simulink library "alfa_wall_out"  (R2018b)
settings: Solver=ode45  StartTime=0.0  StopTime=10.0  RelTol=1e-3  EnableMultiTasking=on
libraries: carnot x2
settings Model: Creator=lena.frank  LastModifiedBy=drhf
settings DataIOCC: LimitDataPoints=on  SaveFormat=Array  SignalLoggingSaveFormat=ModelDataLogs
settings OptimizationCC: ExpressionDepthLimit=2147483647  LifeSpan=inf
settings DebuggingCC: UnderspecifiedInitializationDetection=Classic  MergeDetectMultiDrivingBlocksExec=none  SolverPrmCheckMsg=warning  FcnCallInpInsideContextMsg=warning  StateNameClashWarn=warning  SFUnexpectedBacktrackingDiag=warning  SFNoUnconditionalDefaultTransitionDiag=warning  SFExecutionAtInitializationDiag=none
settings HardwareCC: ProdBitPerPointer=32  ProdBitPerSizeT=32  ProdBitPerPtrDiffT=32  ProdLargestAtomicFloat=None  ProdIntDivRoundTo=Undefined  ProdEndianess=Unspecified  ProdWordSize=32  ProdHWDeviceType=32-bit Generic
settings ModelReferenceCC: PropagateSignalLabelsOutOfModel=off
settings SFSimCC: SimUseLocalCustomCode=off
settings RTWCC: RTWUseLocalCustomCode=off
settings CodeAppCC: StateflowObjectComments=on
settings GRTTargetCC: TargetLangStandard=C89/C90 (ANSI)  GeneratePreprocessorConditionals=Disable all  CombineOutputUpdateFcns=off  GRTInterface=on
settings ConfigComp: CovMetricSettings=dw  CovHtmlReporting=on  CovSaveCumulativeToWorkspaceVar=on  CovSaveSingleToWorkspaceVar=on  CovExternalEMLEnable=off

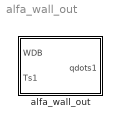
== system alfa_wall_out ==
  alfa_wall_out : Subsystem  mask(ALFA){pos=0, absorption_out=0.4, emission_out=0.7, wallsurface=1}
      mask prompts: pos "Azimut (south = 0, east = -90) in degrees"; absorption_out "Solar absorption outside (0..1)"; emission_out "Longwave emissivity of surface (0..1)"; wallsurface "Wall surface in m²"
      mask help:
      | Convective and radiative HEAT TRANSFER at the WEATHER EXPOSED SURFACE of an OUTER WALL.
      |
      | [W*] : modified weather data, adapted to height over ground,
      | Ts : temperature of outdoor wall surface, °C,
      | qdots : specific heat flow into wall / window construction, W/m^2.
      mask init:
      | if length(pos) == 1
      |     pos = [90  pos 0]; % pos is [inclination azimut rotation]
      | end
      mask Help: web(fullfile(path_carnot('help'),'alfa_wall_out.html'),'-helpbrowser')

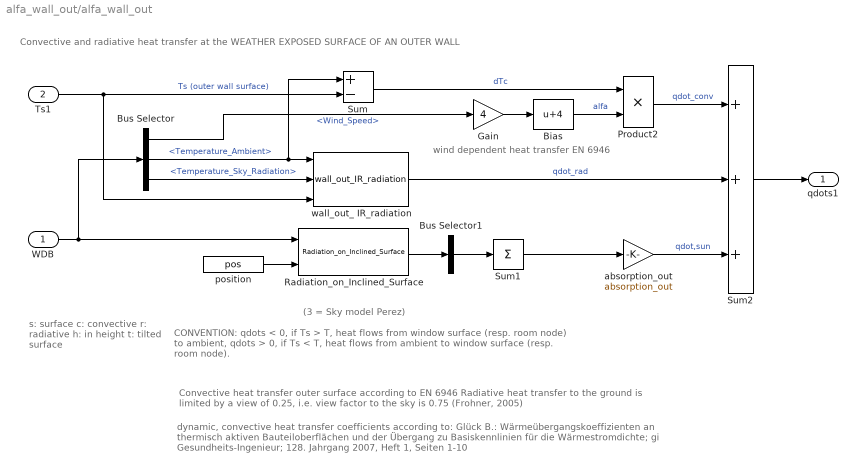
== system alfa_wall_out/alfa_wall_out ==
  note: (3 = Sky model Perez)
  note: wind dependent heat transfer EN 6946
  note: CONVENTION:
      | qdots < 0, if Ts > T, heat flows from window surface (resp. room node) to ambient,
      | qdots > 0, if Ts < T, heat flows from ambient to window surface (resp. room node).
  note: s: surface
      | c: convective
      | r: radiative
      | h: in height
      | t: tilted surface
  note: Convective and radiative heat transfer at the WEATHER EXPOSED SURFACE OF AN OUTER WALL
  note: Convective heat transfer outer surface according to EN 6946
      | Radiative heat transfer to the ground is limited by a view of 0.25, i.e. view factor to the sky is 0.75 (Frohner, 2005)
  note: dynamic, convective heat transfer coefficients according to: Glück B.: Wärmeübergangskoeffizienten an thermisch aktiven Bauteiloberflächen
      | und der Übergang zu Basiskennlinien für die Wärmestromdichte; gi Gesundheits-Ingenieur; 128. Jahrgang 2007, Heft 1, Seiten 1-10
  WDB : Inport
  Ts1 : Inport  Port=2
  Bias : Bias  Bias=4
  Bus Selector : BusSelector  OutputSignals=Wind_Speed,Temperature_Ambient,Temperature_Sky_Radiation
  Bus Selector1 : BusSelector  OutputSignals=Solar_Radiation_direct_surface,Solar_Radiation_diffuse_surface  OutputAsBus=on
  Gain : Gain  Gain=4
  Product2 : Product  SaturateOnIntegerOverflow=on  RndMeth=Zero  InputSameDT=on  OutDataTypeStr=Inherit: Same as first input
  Radiation_on_Inclined_Surface : carnot/Weather/Radiation_on_Inclined_Surface  sky=Perez 1990  reflect=0.2
      settings: SourceProductName=Carnot
  Sum : Sum  Inputs=+-  SaturateOnIntegerOverflow=on  InputSameDT=on  OutDataTypeStr=Inherit: Same as first input
  Sum1 : Sum  Inputs=1  SaturateOnIntegerOverflow=on  InputSameDT=on  OutDataTypeStr=Inherit: Same as first input
  Sum2 : Sum  Inputs=+++  SaturateOnIntegerOverflow=on  InputSameDT=on  OutDataTypeStr=Inherit: Same as first input
  absorption_out : Gain  Gain=absorption_out  SaturateOnIntegerOverflow=on  OutDataTypeStr=Inherit: Same as input  ParamDataTypeStr=Inherit: Same as input
  position : Constant  Value=pos
  wall_out_ IR_radiation : carnot/Basic/Heat_Transfer/wall_out_IR_radiation  SystemSampleTime=-1
      settings: SourceProductName=Carnot
  qdots1 : Outport
  wires:
  position/1 -> Radiation_on_Inclined_Surface/2
  Radiation_on_Inclined_Surface/1 -> Bus Selector1/1
  Bus Selector1/1 -> Sum1/1
  wall_out_ IR_radiation/1 -> Sum2/2  "qdot_rad"
  Product2/1 -> Sum2/1  "qdot_conv"
  absorption_out/1 -> Sum2/3  "qdot,sun"
  Bias/1 -> Product2/2  "alfa"
  Sum1/1 -> absorption_out/1
  Ts1/1 -> Sum/2, wall_out_ IR_radiation/3  "Ts (outer wall surface)"
  Sum2/1 -> qdots1/1
  WDB/1 -> Bus Selector/1, Radiation_on_Inclined_Surface/1
  Sum/1 -> Product2/1  "dTc"
  Bus Selector/2 -> Sum/1, wall_out_ IR_radiation/1  "<Temperature_Ambient>"
  Bus Selector/3 -> wall_out_ IR_radiation/2  "<Temperature_Sky_Radiation>"
  Bus Selector/1 -> Gain/1  "<Wind_Speed>"
  Gain/1 -> Bias/1
